simulink library "Steer_Control_Axle3"  (R2024b)
settings: Solver=VariableStepAuto  StartTime=0.0  StopTime=10.0  RelTol=1e-3
undefined symbols (not defined in the file): Control
Description:
  | Simscape Vehicle Templates Library
  | 
  | Copyright 2018-2024 The MathWorks, Inc.
settings Model: Creator=smiller  LastModifiedBy=smiller
settings ModelReferenceCC: EnableRefExpFcnMdlSchedulingChecks=on
settings RTWCC: GPUComputeCapability=3.5

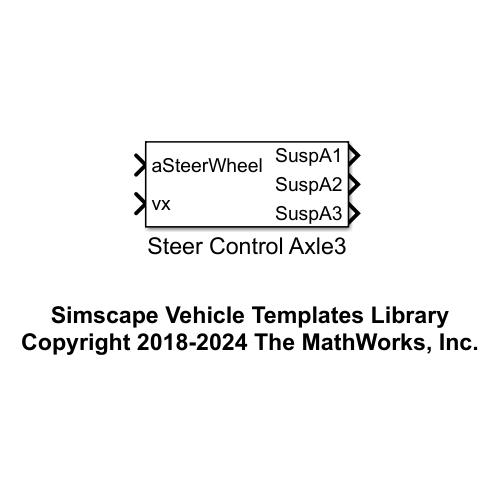
[thumbnail: Simulink's stored preview of the top-level diagram]
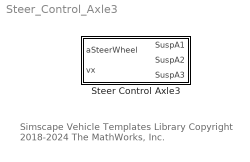
== system Steer_Control_Axle3 ==
  note: Simscape Vehicle Templates Library
      | Copyright 2018-2024 The MathWorks, Inc.
  Steer Control Axle3 : Subsystem  mask(Steer Control, Three Axle){nSteerA2=Control.Default.steer_ratio_axle2, nSteerA3=Control.Default.steer_ratio_axle3}
      mask prompts: nSteerA2 "Axle 2 Steer Ratio"; nSteerA3 "Axle 3 Steer Ratio"
      mask help: Steer control for three-axle vehicles.

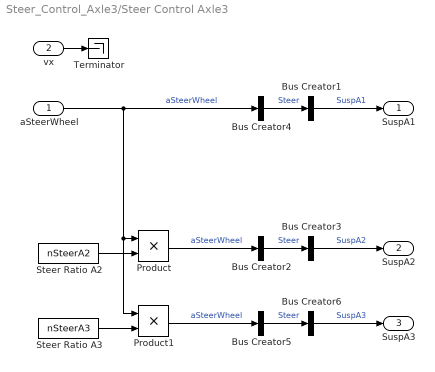
== system Steer_Control_Axle3/Steer Control Axle3 ==
  aSteerWheel : Inport
  vx : Inport  Port=2
  Bus Creator{1..6} (6 alike) : BusCreator  Inputs=1
  Product : Product
  Product1 : Product
  Steer Ratio A2 : Constant  Value=nSteerA2
  Steer Ratio A3 : Constant  Value=nSteerA3
  Terminator : Terminator
  SuspA1 : Outport  VectorParamsAs1DForOutWhenUnconnected=off
  SuspA2 : Outport  Port=2  VectorParamsAs1DForOutWhenUnconnected=off
  SuspA3 : Outport  Port=3  VectorParamsAs1DForOutWhenUnconnected=off
  wires:
  Steer Ratio A3/1 -> Product1/2
  Product1/1 -> Bus Creator5/1  "aSteerWheel"
  Bus Creator6/1 -> SuspA3/1  "SuspA3"
  Bus Creator5/1 -> Bus Creator6/1  "Steer"
  Bus Creator4/1 -> Bus Creator1/1  "Steer"
  Bus Creator2/1 -> Bus Creator3/1  "Steer"
  Bus Creator3/1 -> SuspA2/1  "SuspA2"
  Bus Creator1/1 -> SuspA1/1  "SuspA1"
  aSteerWheel/1 -> Product/1, Product1/1, Bus Creator4/1  "aSteerWheel"
  Product/1 -> Bus Creator2/1  "aSteerWheel"
  vx/1 -> Terminator/1
  Steer Ratio A2/1 -> Product/2
